simulink library "icd"  (Simulink 8.1)
settings: Solver=ode1  StartTime=0.0  StopTime=Inf  FixedStep=0.001  RelTol=1e-3
PostLoadFcn:
  | , if any(exist('dsrtsu_mdlpostloadfcn', 'file') == [2, 3, 6]), try dsrtsu_mdlpostloadfcn('Execute', bdroot); catch fprintf('Error in PostLoadFcn (dsrtsu_mdlpostloadfcn) for model "%s":\n %s\n', bdroot, lasterr); end, end,
undefined symbols (not defined in the file or in its folder): KACC_BrakeToStopDecel_mps2, KACC_BrakeToStopMCAddedDecel_mps2
settings Model: DSRTSU_INTERNAL_RTI_VER=450  DSRTSU_INTERNAL_RTI_TYPE=rti1401  Creator=AT015555  LastModifiedBy=AT015555

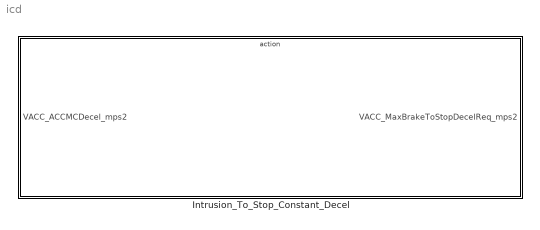
== system icd ==
  Intrusion_To_Stop_Constant_Decel : Subsystem  TreatAsAtomicUnit=on

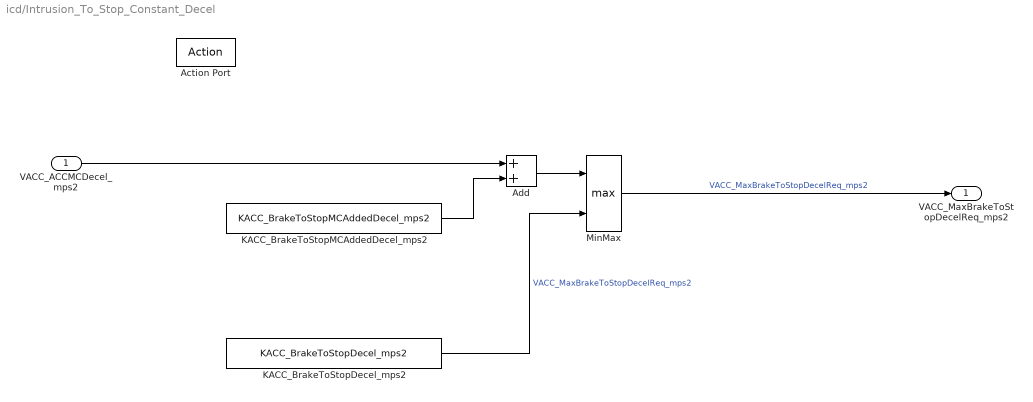
== system icd/Intrusion_To_Stop_Constant_Decel ==
  VACC_ACCMCDecel_mps2 : Inport
  Action Port : ActionPort
  Add : Sum
  KACC_BrakeToStopDecel_mps2 : Constant  Value=KACC_BrakeToStopDecel_mps2
  KACC_BrakeToStopMCAddedDecel_mps2 : Constant  Value=KACC_BrakeToStopMCAddedDecel_mps2  OutDataTypeStr=single
  MinMax : MinMax  Function=max  Inputs=2
  VACC_MaxBrakeToStopDecelReq_mps2 : Outport
  wires:
  KACC_BrakeToStopDecel_mps2/1 -> MinMax/2  "VACC_MaxBrakeToStopDecelReq_mps2"
  Add/1 -> MinMax/1
  KACC_BrakeToStopMCAddedDecel_mps2/1 -> Add/2
  VACC_ACCMCDecel_mps2/1 -> Add/1
  MinMax/1 -> VACC_MaxBrakeToStopDecelReq_mps2/1  "VACC_MaxBrakeToStopDecelReq_mps2"
